simulink model "test_drop_mech"  (Simulink 7.6)
settings: Solver=FixedStepDiscrete  StartTime=0.0  StopTime=0  RelTol=1e-3
undefined symbols (not defined in the file or in its folder): black_al, black_au, black_bl, black_bu, blue_al, blue_au, blue_bl, blue_bu, Down_Camera_Dimensions, gray, green_al, green_au, green_bl, green_bu, Iter_Segment_Thresh, jet, orange_al, orange_au, orange_bl, orange_bu, Rec, red_al, red_au, red_bl, red_bu, Scale_Down_B, Scale_Down_G, Scale_Down_H, Scale_Down_R, Scale_Down_S, Scale_Down_V, SDTV, white_al, white_au, white_bl, white_bu, yellow_al, yellow_au, yellow_bl, yellow_bu
libraries: vipconversions x8, vipgeotforms x6, vipsnks x4, viptextngfix x2, vipsrcs x1
(part 1 of 2)
settings Model: Creator=Thing 1  LastModifiedBy=auvt
settings RTWCC: TargetLang=C++

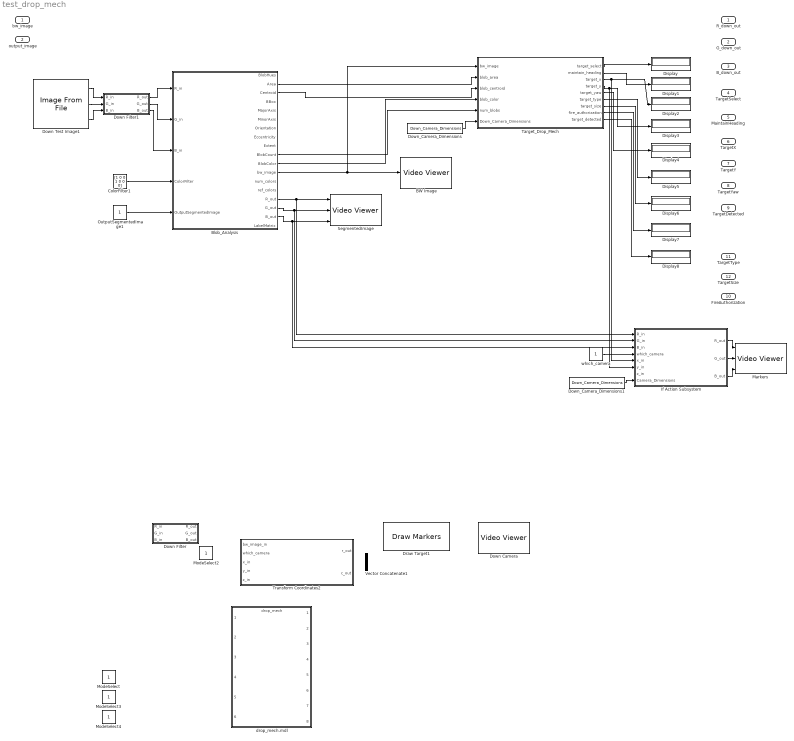
== system test_drop_mech ==
  bw_image : Inport
  output_image : Inport  Port=2
  BW Image : vipsnks/Video Viewer  DialogControllerArgs=DataTag1  inputType=Obsolete7b  imagePorts=One multidimensional signal  useColorMap=off  colormapValue=gray(256)  specRange=off  minInputVal=0  maxInputVal=255  FigPos=[5 861 410 300]  AxisZoom=on  trueSizedOnce=off  OpenAtMdlStart=on
  Blob_Analysis : Subsystem
  ColorFilter1 : Constant  Value=[1 0 0 1 0 0 0]  SampleTime=-1
  Display{,1..8} (9 alike) : Display
  Down Camera : vipsnks/Video Viewer  DialogControllerArgs=DataTag9  inputType=Obsolete7b  imagePorts=Separate color signals  useColorMap=off  colormapValue=jet(256)  specRange=off  minInputVal=0  maxInputVal=255  FigPos=[970 679 274 199]  AxisZoom=on  trueSizedOnce=off  OpenAtMdlStart=on
  Down Filter : Subsystem
  Down Filter1 : Subsystem
  Down Test Image1 : vipsrcs/Image From File  Tag=vipblks_nd  DialogController=vipDDGCreate  DialogControllerArgs=DataTag10  SystemSampleTime=-1  FileName=/home/auvt/auvc/src/vision/Test_Images/drop1.png  imagePorts=Separate color signals  Ts=-1  ImageDataType=double  Signed=on  WordLength=16  sdImageDataType=uint(8)  FractionLengthMode=User-defined  FractionLength=15  OutPortLabels=R|G|B
  Down_Camera_Dimensions : Constant  Value=Down_Camera_Dimensions  SampleTime=-1
  Down_Camera_Dimensions1 : Constant  Value=Down_Camera_Dimensions  SampleTime=-1
  Draw Target1 : viptextngfix/Draw Markers  DialogController=vipDDGCreate  DialogControllerArgs=DataTag11  shape=X-mark  size=7  fill=off  fillClrSource=Specify via dialog  display=User-specified value  intensity=200  color=[0 0 0]  opacity=0.6  viewport=Entire image  antialiasing=off  inType=Obsolete  imagePorts=Separate color signals  prodOutputMode=Binary point scaling  prodOutputWordLength=32  prodOutputFracLength=14  memoryMode=Specify word length  memoryWordLength=16  memoryFracLength=15  roundingMode=Floor  overflowMode=off
  If Action Subsystem : Subsystem  TreatAsAtomicUnit=on
  Markers : vipsnks/Video Viewer  DialogControllerArgs=DataTag14  inputType=Obsolete7b  imagePorts=Separate color signals  useColorMap=off  colormapValue=gray(256)  specRange=off  minInputVal=0  maxInputVal=255  FigPos=[421 436 410 300]  AxisZoom=on  trueSizedOnce=off  OpenAtMdlStart=on
  ModeSelect{,2..4} (4 alike) : Constant  SampleTime=-1
  OutputSegmentedImage1 : Constant  SampleTime=-1
  SegmentedImage : vipsnks/Video Viewer  DialogControllerArgs=DataTag16  inputType=Obsolete7b  imagePorts=Separate color signals  useColorMap=off  colormapValue=gray(256)  specRange=off  minInputVal=0  maxInputVal=255  FigPos=[5 436 410 300]  AxisZoom=on  trueSizedOnce=off  OpenAtMdlStart=on
  Target_Drop_Mech : Stateflow chart  TreatAsAtomicUnit=on  SystemSampleTime=[1/30 0]
  Transform Coordinates2 : Stateflow chart  TreatAsAtomicUnit=on  SystemSampleTime=[1/30 0]
  Vector Concatenate1 : Concatenate  Mode=Multidimensional array
  drop_mech.mdl : ModelReference  ModelNameDialog=drop_mech  SimulationMode=Accelerator  ModelReferenceVersion=1.17  CopyOfModelName=drop_mech
  which_camera : Constant  SampleTime=-1
  R_down_out : Outport  OutDataTypeStr=double
  G_down_out : Outport  Port=2  OutDataTypeStr=double
  B_down_out : Outport  Port=3  OutDataTypeStr=double
  TargetSelect : Outport  Port=4  OutDataTypeStr=double
  MaintainHeading : Outport  Port=5  OutDataTypeStr=double
  TargetX : Outport  Port=6  OutDataTypeStr=double
  TargetY : Outport  Port=7  OutDataTypeStr=double
  TargetYaw : Outport  Port=8  OutDataTypeStr=double
  TargetDetected : Outport  Port=9  OutDataTypeStr=double
  FireAuthorization : Outport  Port=10  OutDataTypeStr=double
  TargetType : Outport  Port=11  OutDataTypeStr=double
  TargetSize : Outport  Port=12  OutDataTypeStr=double
  wires:
  OutputSegmentedImage1/1 -> Blob_Analysis/5(OutputSegmentedImage)
  ColorFilter1/1 -> Blob_Analysis/4(ColorFilter)
  Down Test Image1/1 -> Down Filter1/1(R_in)
  Down Test Image1/2 -> Down Filter1/2(G_in)
  Down Test Image1/3 -> Down Filter1/3(B_in)
  Down Filter1/1(R_out) -> Blob_Analysis/1(R_in)
  Down Filter1/2(G_out) -> Blob_Analysis/2(G_in)
  Down Filter1/3(B_out) -> Blob_Analysis/3(B_in)
  Blob_Analysis/15(R_out) -> If Action Subsystem/1(R_in), SegmentedImage/1
  Blob_Analysis/16(G_out) -> If Action Subsystem/2(G_in), SegmentedImage/2
  Blob_Analysis/17(B_out) -> If Action Subsystem/3(B_in), SegmentedImage/3
  Blob_Analysis/3(Centroid) -> Target_Drop_Mech/3(blob_centroid)
  Blob_Analysis/12(bw_image) -> BW Image/1, Target_Drop_Mech/1(bw_image)
  Blob_Analysis/2(Area) -> Target_Drop_Mech/2(blob_area)
  Blob_Analysis/11(BlobColor) -> Target_Drop_Mech/4(blob_color)
  Blob_Analysis/10(BlobCount) -> Target_Drop_Mech/5(num_blobs)
  Down_Camera_Dimensions/1 -> Target_Drop_Mech/6(Down_Camera_Dimensions)
  Target_Drop_Mech/1(target_select) -> Display/1
  Target_Drop_Mech/2(maintain_heading) -> Display1/1
  Target_Drop_Mech/3(target_x) -> Display2/1, If Action Subsystem/5(x_in)
  Target_Drop_Mech/4(target_y) -> Display3/1, If Action Subsystem/6(y_in)
  Target_Drop_Mech/5(target_yaw) -> Display4/1
  Target_Drop_Mech/6(target_type) -> Display5/1
  Target_Drop_Mech/7(target_size) -> Display6/1
  which_camera/1 -> If Action Subsystem/4(which_camera)
  If Action Subsystem/1(R_out) -> Markers/1
  If Action Subsystem/2(G_out) -> Markers/2
  If Action Subsystem/3(B_out) -> Markers/3
  Down_Camera_Dimensions1/1 -> If Action Subsystem/8(Camera_Dimensions)
  Target_Drop_Mech/8(fire_authorization) -> Display7/1
  Target_Drop_Mech/9(target_detected) -> Display8/1

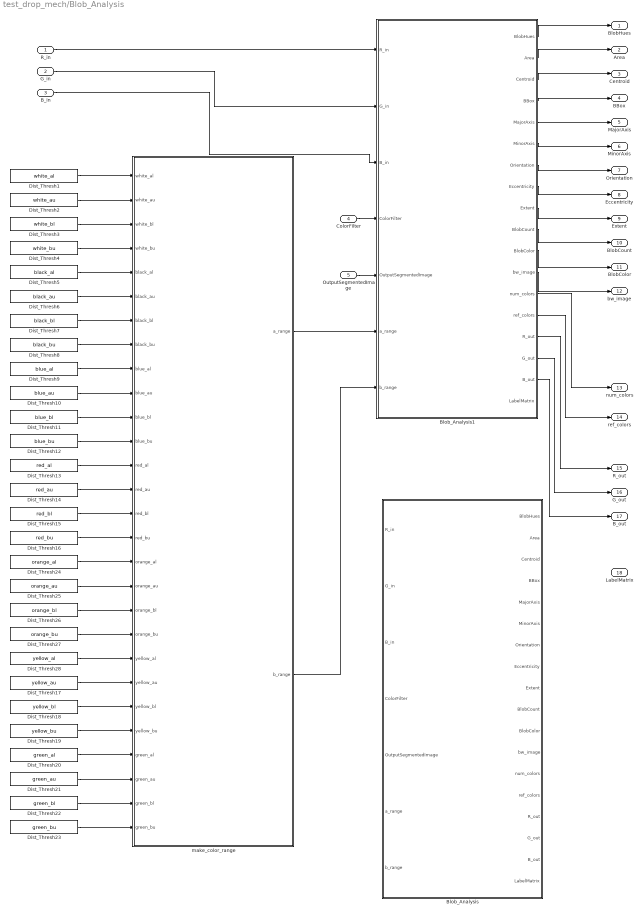
== system test_drop_mech/Blob_Analysis ==
  R_in : Inport
  G_in : Inport  Port=2
  B_in : Inport  Port=3
  ColorFilter : Inport  Port=4
  OutputSegmentedImage : Inport  Port=5
  Blob_Analysis : Subsystem  TreatAsAtomicUnit=on
  Blob_Analysis1 : Subsystem  TreatAsAtomicUnit=on
  Dist_Thresh1 : Constant  Value=white_al  SampleTime=-1
  Dist_Thresh10 : Constant  Value=blue_au  SampleTime=-1
  Dist_Thresh11 : Constant  Value=blue_bl  SampleTime=-1
  Dist_Thresh12 : Constant  Value=blue_bu  SampleTime=-1
  Dist_Thresh13 : Constant  Value=red_al  SampleTime=-1
  Dist_Thresh14 : Constant  Value=red_au  SampleTime=-1
  Dist_Thresh15 : Constant  Value=red_bl  SampleTime=-1
  Dist_Thresh16 : Constant  Value=red_bu  SampleTime=-1
  Dist_Thresh17 : Constant  Value=yellow_au  SampleTime=-1
  Dist_Thresh18 : Constant  Value=yellow_bl  SampleTime=-1
  Dist_Thresh19 : Constant  Value=yellow_bu  SampleTime=-1
  Dist_Thresh2 : Constant  Value=white_au  SampleTime=-1
  Dist_Thresh20 : Constant  Value=green_al  SampleTime=-1
  Dist_Thresh21 : Constant  Value=green_au  SampleTime=-1
  Dist_Thresh22 : Constant  Value=green_bl  SampleTime=-1
  Dist_Thresh23 : Constant  Value=green_bu  SampleTime=-1
  Dist_Thresh24 : Constant  Value=orange_al  SampleTime=-1
  Dist_Thresh25 : Constant  Value=orange_au  SampleTime=-1
  Dist_Thresh26 : Constant  Value=orange_bl  SampleTime=-1
  Dist_Thresh27 : Constant  Value=orange_bu  SampleTime=-1
  Dist_Thresh28 : Constant  Value=yellow_al  SampleTime=-1
  Dist_Thresh3 : Constant  Value=white_bl  SampleTime=-1
  Dist_Thresh4 : Constant  Value=white_bu  SampleTime=-1
  Dist_Thresh5 : Constant  Value=black_al  SampleTime=-1
  Dist_Thresh6 : Constant  Value=black_au  SampleTime=-1
  Dist_Thresh7 : Constant  Value=black_bl  SampleTime=-1
  Dist_Thresh8 : Constant  Value=black_bu  SampleTime=-1
  Dist_Thresh9 : Constant  Value=blue_al  SampleTime=-1
  make_color_range : Stateflow chart  TreatAsAtomicUnit=on
  BlobHues : Outport
  Area : Outport  Port=2
  Centroid : Outport  Port=3
  BBox : Outport  Port=4
  MajorAxis : Outport  Port=5
  MinorAxis : Outport  Port=6
  Orientation : Outport  Port=7
  Eccentricity : Outport  Port=8
  Extent : Outport  Port=9
  BlobCount : Outport  Port=10
  BlobColor : Outport  Port=11
  bw_image : Outport  Port=12
  num_colors : Outport  Port=13
  ref_colors : Outport  Port=14
  R_out : Outport  Port=15
  G_out : Outport  Port=16
  B_out : Outport  Port=17
  LabelMatrix : Outport  Port=18
  wires:
  ColorFilter/1 -> Blob_Analysis1/4(ColorFilter)
  OutputSegmentedImage/1 -> Blob_Analysis1/5(OutputSegmentedImage)
  make_color_range/2(b_range) -> Blob_Analysis1/7(b_range)
  make_color_range/1(a_range) -> Blob_Analysis1/6(a_range)
  B_in/1 -> Blob_Analysis1/3(B_in)
  G_in/1 -> Blob_Analysis1/2(G_in)
  R_in/1 -> Blob_Analysis1/1(R_in)
  Dist_Thresh7/1 -> make_color_range/7(black_bl)
  Dist_Thresh6/1 -> make_color_range/6(black_au)
  Dist_Thresh5/1 -> make_color_range/5(black_al)
  Dist_Thresh4/1 -> make_color_range/4(white_bu)
  Dist_Thresh3/1 -> make_color_range/3(white_bl)
  Dist_Thresh2/1 -> make_color_range/2(white_au)
  Dist_Thresh8/1 -> make_color_range/8(black_bu)
  Dist_Thresh9/1 -> make_color_range/9(blue_al)
  Dist_Thresh10/1 -> make_color_range/10(blue_au)
  Dist_Thresh11/1 -> make_color_range/11(blue_bl)
  Dist_Thresh12/1 -> make_color_range/12(blue_bu)
  Dist_Thresh13/1 -> make_color_range/13(red_al)
  Dist_Thresh14/1 -> make_color_range/14(red_au)
  Dist_Thresh15/1 -> make_color_range/15(red_bl)
  Dist_Thresh16/1 -> make_color_range/16(red_bu)
  Dist_Thresh24/1 -> make_color_range/17(orange_al)
  Dist_Thresh25/1 -> make_color_range/18(orange_au)
  Dist_Thresh26/1 -> make_color_range/19(orange_bl)
  Dist_Thresh27/1 -> make_color_range/20(orange_bu)
  Dist_Thresh21/1 -> make_color_range/26(green_au)
  Dist_Thresh28/1 -> make_color_range/21(yellow_al)
  Dist_Thresh17/1 -> make_color_range/22(yellow_au)
  Dist_Thresh20/1 -> make_color_range/25(green_al)
  Dist_Thresh19/1 -> make_color_range/24(yellow_bu)
  Dist_Thresh18/1 -> make_color_range/23(yellow_bl)
  Dist_Thresh1/1 -> make_color_range/1(white_al)
  Dist_Thresh22/1 -> make_color_range/27(green_bl)
  Dist_Thresh23/1 -> make_color_range/28(green_bu)
  Blob_Analysis1/1(BlobHues) -> BlobHues/1
  Blob_Analysis1/2(Area) -> Area/1
  Blob_Analysis1/3(Centroid) -> Centroid/1
  Blob_Analysis1/4(BBox) -> BBox/1
  Blob_Analysis1/5(MajorAxis) -> MajorAxis/1
  Blob_Analysis1/6(MinorAxis) -> MinorAxis/1
  Blob_Analysis1/7(Orientation) -> Orientation/1
  Blob_Analysis1/8(Eccentricity) -> Eccentricity/1
  Blob_Analysis1/9(Extent) -> Extent/1
  Blob_Analysis1/10(BlobCount) -> BlobCount/1
  Blob_Analysis1/11(BlobColor) -> BlobColor/1
  Blob_Analysis1/12(bw_image) -> bw_image/1
  Blob_Analysis1/13(num_colors) -> num_colors/1
  Blob_Analysis1/14(ref_colors) -> ref_colors/1
  Blob_Analysis1/15(R_out) -> R_out/1
  Blob_Analysis1/16(G_out) -> G_out/1
  Blob_Analysis1/17(B_out) -> B_out/1

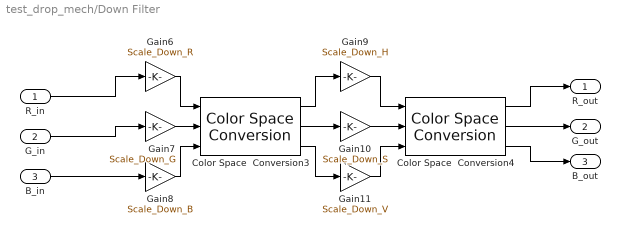
== system test_drop_mech/Down Filter ==
  R_in : Inport  PortDimensions=Down_Camera_Dimensions
  G_in : Inport  Port=2  PortDimensions=Down_Camera_Dimensions
  B_in : Inport  Port=3  PortDimensions=Down_Camera_Dimensions
  Color Space  Conversion3 : vipconversions/Color Space  Conversion  conversion=Obsolete  conversionActive=R'G'B' to HSV  wp_str=D50  rec=Rec. 601 (SDTV)  sys=1125/60/2:1  imagePorts=Separate color signals
  Color Space  Conversion4 : vipconversions/Color Space  Conversion  conversion=Obsolete  conversionActive=HSV to R'G'B'  wp_str=D50  rec=Rec. 601 (SDTV)  sys=1125/60/2:1  imagePorts=Separate color signals
  Gain10 : Gain  Gain=Scale_Down_S
  Gain11 : Gain  Gain=Scale_Down_V
  Gain6 : Gain  Gain=Scale_Down_R
  Gain7 : Gain  Gain=Scale_Down_G
  Gain8 : Gain  Gain=Scale_Down_B
  Gain9 : Gain  Gain=Scale_Down_H
  R_out : Outport  OutDataTypeStr=double
  G_out : Outport  Port=2  OutDataTypeStr=double
  B_out : Outport  Port=3  OutDataTypeStr=double
  wires:
  Gain6/1 -> Color Space  Conversion3/1
  Gain7/1 -> Color Space  Conversion3/2
  Gain8/1 -> Color Space  Conversion3/3
  Color Space  Conversion3/1 -> Gain9/1
  Color Space  Conversion3/2 -> Gain10/1
  Color Space  Conversion3/3 -> Gain11/1
  Gain9/1 -> Color Space  Conversion4/1
  Gain10/1 -> Color Space  Conversion4/2
  Gain11/1 -> Color Space  Conversion4/3
  R_in/1 -> Gain6/1
  G_in/1 -> Gain7/1
  B_in/1 -> Gain8/1
  Color Space  Conversion4/1 -> R_out/1
  Color Space  Conversion4/2 -> G_out/1
  Color Space  Conversion4/3 -> B_out/1

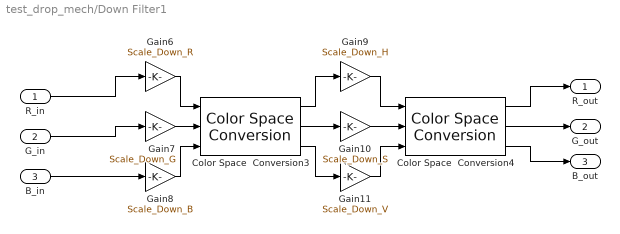
== system test_drop_mech/Down Filter1 ==
  R_in : Inport  PortDimensions=Down_Camera_Dimensions
  G_in : Inport  Port=2  PortDimensions=Down_Camera_Dimensions
  B_in : Inport  Port=3  PortDimensions=Down_Camera_Dimensions
  Color Space  Conversion3 : vipconversions/Color Space  Conversion  conversion=Obsolete  conversionActive=R'G'B' to HSV  wp_str=D50  rec=Rec. 601 (SDTV)  sys=1125/60/2:1  imagePorts=Separate color signals
  Color Space  Conversion4 : vipconversions/Color Space  Conversion  conversion=Obsolete  conversionActive=HSV to R'G'B'  wp_str=D50  rec=Rec. 601 (SDTV)  sys=1125/60/2:1  imagePorts=Separate color signals
  Gain10 : Gain  Gain=Scale_Down_S
  Gain11 : Gain  Gain=Scale_Down_V
  Gain6 : Gain  Gain=Scale_Down_R
  Gain7 : Gain  Gain=Scale_Down_G
  Gain8 : Gain  Gain=Scale_Down_B
  Gain9 : Gain  Gain=Scale_Down_H
  R_out : Outport  OutDataTypeStr=double
  G_out : Outport  Port=2  OutDataTypeStr=double
  B_out : Outport  Port=3  OutDataTypeStr=double
  wires:
  Gain6/1 -> Color Space  Conversion3/1
  Gain7/1 -> Color Space  Conversion3/2
  Gain8/1 -> Color Space  Conversion3/3
  Color Space  Conversion3/1 -> Gain9/1
  Color Space  Conversion3/2 -> Gain10/1
  Color Space  Conversion3/3 -> Gain11/1
  Gain9/1 -> Color Space  Conversion4/1
  Gain10/1 -> Color Space  Conversion4/2
  Gain11/1 -> Color Space  Conversion4/3
  R_in/1 -> Gain6/1
  G_in/1 -> Gain7/1
  B_in/1 -> Gain8/1
  Color Space  Conversion4/1 -> R_out/1
  Color Space  Conversion4/2 -> G_out/1
  Color Space  Conversion4/3 -> B_out/1

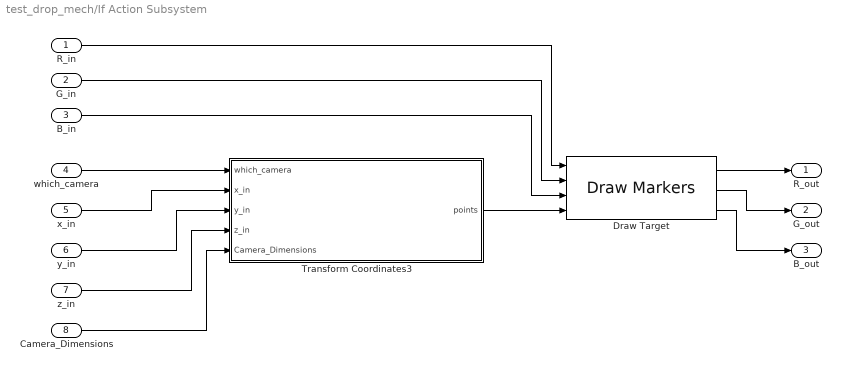
== system test_drop_mech/If Action Subsystem ==
  R_in : Inport
  G_in : Inport  Port=2
  B_in : Inport  Port=3
  which_camera : Inport  Port=4
  x_in : Inport  Port=5
  y_in : Inport  Port=6
  z_in : Inport  Port=7
  Camera_Dimensions : Inport  Port=8
  Draw Target : viptextngfix/Draw Markers  DialogController=vipDDGCreate  DialogControllerArgs=DataTag12  shape=X-mark  size=7  fill=off  fillClrSource=Specify via dialog  display=User-specified value  intensity=200  color=[1 1 0]  opacity=0.6  viewport=Entire image  antialiasing=off  inType=Obsolete  imagePorts=Separate color signals  prodOutputMode=Binary point scaling  prodOutputWordLength=32  prodOutputFracLength=14  memoryMode=Specify word length  memoryWordLength=16  memoryFracLength=15  roundingMode=Floor  overflowMode=off
  Transform Coordinates3 : Stateflow chart  TreatAsAtomicUnit=on
  R_out : Outport  OutDataTypeStr=double
  G_out : Outport  Port=2  OutDataTypeStr=double
  B_out : Outport  Port=3  OutDataTypeStr=double
  wires:
  which_camera/1 -> Transform Coordinates3/1(which_camera)
  x_in/1 -> Transform Coordinates3/2(x_in)
  y_in/1 -> Transform Coordinates3/3(y_in)
  z_in/1 -> Transform Coordinates3/4(z_in)
  Camera_Dimensions/1 -> Transform Coordinates3/5(Camera_Dimensions)
  Draw Target/1 -> R_out/1
  Draw Target/2 -> G_out/1
  Draw Target/3 -> B_out/1
  R_in/1 -> Draw Target/1
  G_in/1 -> Draw Target/2
  B_in/1 -> Draw Target/3
  Transform Coordinates3/1(points) -> Draw Target/4

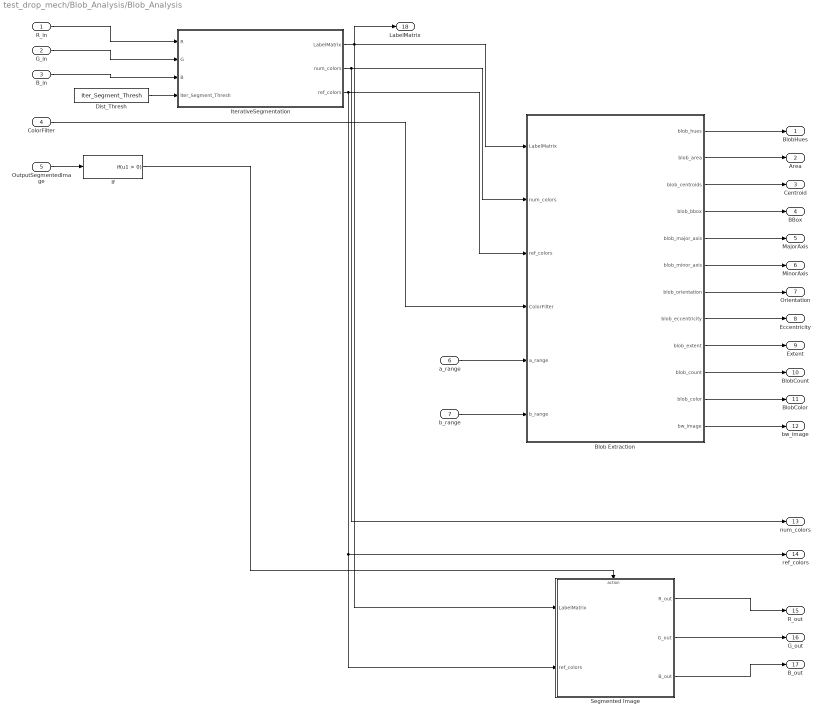
== system test_drop_mech/Blob_Analysis/Blob_Analysis ==
  R_in : Inport
  G_in : Inport  Port=2
  B_in : Inport  Port=3
  ColorFilter : Inport  Port=4
  OutputSegmentedImage : Inport  Port=5
  a_range : Inport  Port=6
  b_range : Inport  Port=7
  Blob Extraction : Stateflow chart  TreatAsAtomicUnit=on
  Dist_Thresh : Constant  Value=Iter_Segment_Thresh  SampleTime=-1
  If : If  ShowElse=off
  IterativeSegmentation : Subsystem
      settings: UndoDeleteFcn=Stateflow.SLINSF.SimulinkMan.restorePreDeleteFcn  PreDeleteFcn=Stateflow.SLINSF.SimulinkMan.removePreDeleteFcn
  Segmented Image : Subsystem  TreatAsAtomicUnit=on
  BlobHues : Outport
  Area : Outport  Port=2
  Centroid : Outport  Port=3
  BBox : Outport  Port=4
  MajorAxis : Outport  Port=5
  MinorAxis : Outport  Port=6
  Orientation : Outport  Port=7
  Eccentricity : Outport  Port=8
  Extent : Outport  Port=9
  BlobCount : Outport  Port=10
  BlobColor : Outport  Port=11
  bw_image : Outport  Port=12
  num_colors : Outport  Port=13
  ref_colors : Outport  Port=14
  R_out : Outport  Port=15
  G_out : Outport  Port=16
  B_out : Outport  Port=17
  LabelMatrix : Outport  Port=18
  wires:
  Blob Extraction/11(blob_color) -> BlobColor/1
  Segmented Image/3(B_out) -> B_out/1
  Segmented Image/2(G_out) -> G_out/1
  Segmented Image/1(R_out) -> R_out/1
  OutputSegmentedImage/1 -> If/1
  If/1 -> Segmented Image/Action
  B_in/1 -> IterativeSegmentation/3(B)
  G_in/1 -> IterativeSegmentation/2(G)
  R_in/1 -> IterativeSegmentation/1(R)
  Dist_Thresh/1 -> IterativeSegmentation/4(Iter_Segment_Thresh)
  IterativeSegmentation/3(ref_colors) -> ref_colors/1, Segmented Image/2(ref_colors), Blob Extraction/3(ref_colors)
  IterativeSegmentation/2(num_colors) -> num_colors/1, Blob Extraction/2(num_colors)
  IterativeSegmentation/1(LabelMatrix) -> LabelMatrix/1, Segmented Image/1(LabelMatrix), Blob Extraction/1(LabelMatrix)
  b_range/1 -> Blob Extraction/6(b_range)
  a_range/1 -> Blob Extraction/5(a_range)
  ColorFilter/1 -> Blob Extraction/4(ColorFilter)
  Blob Extraction/1(blob_hues) -> BlobHues/1
  Blob Extraction/2(blob_area) -> Area/1
  Blob Extraction/3(blob_centroids) -> Centroid/1
  Blob Extraction/4(blob_bbox) -> BBox/1
  Blob Extraction/5(blob_major_axis) -> MajorAxis/1
  Blob Extraction/6(blob_minor_axis) -> MinorAxis/1
  Blob Extraction/7(blob_orientation) -> Orientation/1
  Blob Extraction/8(blob_eccentricity) -> Eccentricity/1
  Blob Extraction/9(blob_extent) -> Extent/1
  Blob Extraction/10(blob_count) -> BlobCount/1
  Blob Extraction/12(bw_image) -> bw_image/1

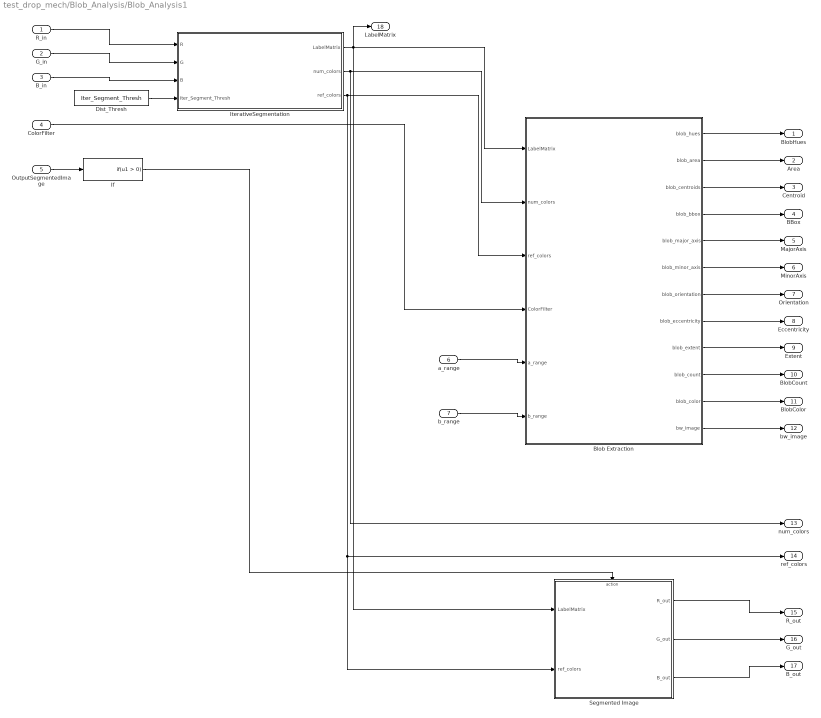
== system test_drop_mech/Blob_Analysis/Blob_Analysis1 ==
  R_in : Inport
  G_in : Inport  Port=2
  B_in : Inport  Port=3
  ColorFilter : Inport  Port=4
  OutputSegmentedImage : Inport  Port=5
  a_range : Inport  Port=6
  b_range : Inport  Port=7
  Blob Extraction : Stateflow chart  TreatAsAtomicUnit=on
  Dist_Thresh : Constant  Value=Iter_Segment_Thresh  SampleTime=-1
  If : If  ShowElse=off
  IterativeSegmentation : Subsystem
      settings: UndoDeleteFcn=Stateflow.SLINSF.SimulinkMan.restorePreDeleteFcn  PreDeleteFcn=Stateflow.SLINSF.SimulinkMan.removePreDeleteFcn
  Segmented Image : Subsystem  TreatAsAtomicUnit=on
  BlobHues : Outport
  Area : Outport  Port=2
  Centroid : Outport  Port=3
  BBox : Outport  Port=4
  MajorAxis : Outport  Port=5
  MinorAxis : Outport  Port=6
  Orientation : Outport  Port=7
  Eccentricity : Outport  Port=8
  Extent : Outport  Port=9
  BlobCount : Outport  Port=10
  BlobColor : Outport  Port=11
  bw_image : Outport  Port=12
  num_colors : Outport  Port=13
  ref_colors : Outport  Port=14
  R_out : Outport  Port=15
  G_out : Outport  Port=16
  B_out : Outport  Port=17
  LabelMatrix : Outport  Port=18
  wires:
  Blob Extraction/12(bw_image) -> bw_image/1
  Blob Extraction/10(blob_count) -> BlobCount/1
  Blob Extraction/9(blob_extent) -> Extent/1
  Blob Extraction/8(blob_eccentricity) -> Eccentricity/1
  Blob Extraction/7(blob_orientation) -> Orientation/1
  Blob Extraction/6(blob_minor_axis) -> MinorAxis/1
  Blob Extraction/5(blob_major_axis) -> MajorAxis/1
  Blob Extraction/4(blob_bbox) -> BBox/1
  Blob Extraction/3(blob_centroids) -> Centroid/1
  Blob Extraction/2(blob_area) -> Area/1
  Blob Extraction/1(blob_hues) -> BlobHues/1
  ColorFilter/1 -> Blob Extraction/4(ColorFilter)
  a_range/1 -> Blob Extraction/5(a_range)
  b_range/1 -> Blob Extraction/6(b_range)
  IterativeSegmentation/1(LabelMatrix) -> Blob Extraction/1(LabelMatrix), Segmented Image/1(LabelMatrix), LabelMatrix/1
  IterativeSegmentation/2(num_colors) -> Blob Extraction/2(num_colors), num_colors/1
  IterativeSegmentation/3(ref_colors) -> Blob Extraction/3(ref_colors), Segmented Image/2(ref_colors), ref_colors/1
  Dist_Thresh/1 -> IterativeSegmentation/4(Iter_Segment_Thresh)
  R_in/1 -> IterativeSegmentation/1(R)
  G_in/1 -> IterativeSegmentation/2(G)
  B_in/1 -> IterativeSegmentation/3(B)
  If/1 -> Segmented Image/Action
  OutputSegmentedImage/1 -> If/1
  Segmented Image/1(R_out) -> R_out/1
  Segmented Image/2(G_out) -> G_out/1
  Segmented Image/3(B_out) -> B_out/1
  Blob Extraction/11(blob_color) -> BlobColor/1

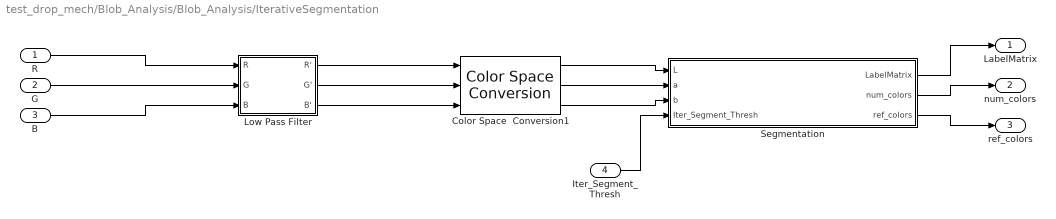
== system test_drop_mech/Blob_Analysis/Blob_Analysis/IterativeSegmentation ==
  R : Inport
  G : Inport  Port=2
  B : Inport  Port=3
  Iter_Segment_Thresh : Inport  Port=4
  Color Space  Conversion1 : vipconversions/Color Space  Conversion  conversion=Obsolete  conversionActive=sR'G'B' to L*a*b*  wp_str=D50  rec=Rec. 601 (SDTV)  sys=1125/60/2:1  imagePorts=Separate color signals
  Low Pass Filter : Subsystem
  Segmentation : Subsystem
  LabelMatrix : Outport
  num_colors : Outport  Port=2
  ref_colors : Outport  Port=3
  wires:
  Iter_Segment_Thresh/1 -> Segmentation/4(Iter_Segment_Thresh)
  Segmentation/3(ref_colors) -> ref_colors/1
  Segmentation/2(num_colors) -> num_colors/1
  Segmentation/1(LabelMatrix) -> LabelMatrix/1
  B/1 -> Low Pass Filter/3(B)
  G/1 -> Low Pass Filter/2(G)
  R/1 -> Low Pass Filter/1(R)
  Color Space  Conversion1/1 -> Segmentation/1(L)
  Color Space  Conversion1/2 -> Segmentation/2(a)
  Color Space  Conversion1/3 -> Segmentation/3(b)
  Low Pass Filter/1(R') -> Color Space  Conversion1/1
  Low Pass Filter/2(G') -> Color Space  Conversion1/2
  Low Pass Filter/3(B') -> Color Space  Conversion1/3

== system test_drop_mech/Blob_Analysis/Blob_Analysis/Segmented Image ==
  LabelMatrix : Inport
  ref_colors : Inport  Port=2
  Action Port : ActionPort
  Color Space  Conversion : vipconversions/Color Space  Conversion  conversion=Obsolete  conversionActive=L*a*b* to sR'G'B'  wp_str=D65  rec=Rec. 601 (SDTV)  sys=1125/60/2:1  imagePorts=Separate color signals
  Display Image : Stateflow chart  TreatAsAtomicUnit=on
  R_out : Outport
  G_out : Outport  Port=2
  B_out : Outport  Port=3
  wires:
  Color Space  Conversion/3 -> B_out/1
  Color Space  Conversion/2 -> G_out/1
  Color Space  Conversion/1 -> R_out/1
  Display Image/3(b) -> Color Space  Conversion/3
  Display Image/2(a) -> Color Space  Conversion/2
  Display Image/1(L) -> Color Space  Conversion/1
  ref_colors/1 -> Display Image/2(ref_colors)
  LabelMatrix/1 -> Display Image/1(LabelMatrix)

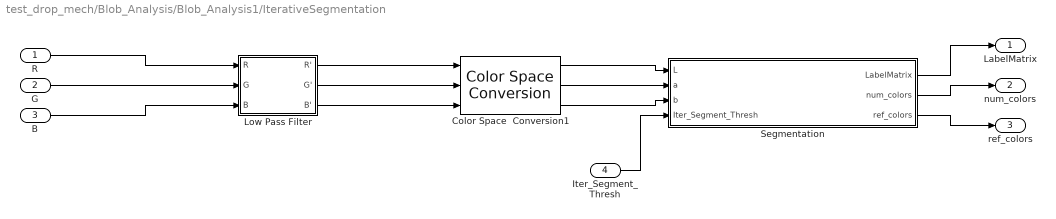
== system test_drop_mech/Blob_Analysis/Blob_Analysis1/IterativeSegmentation ==
  R : Inport
  G : Inport  Port=2
  B : Inport  Port=3
  Iter_Segment_Thresh : Inport  Port=4
  Color Space  Conversion1 : vipconversions/Color Space  Conversion  conversion=Obsolete  conversionActive=sR'G'B' to L*a*b*  wp_str=D50  rec=Rec. 601 (SDTV)  sys=1125/60/2:1  imagePorts=Separate color signals
  Low Pass Filter : Subsystem
  Segmentation : Subsystem
  LabelMatrix : Outport
  num_colors : Outport  Port=2
  ref_colors : Outport  Port=3
  wires:
  Low Pass Filter/3(B') -> Color Space  Conversion1/3
  Low Pass Filter/2(G') -> Color Space  Conversion1/2
  Low Pass Filter/1(R') -> Color Space  Conversion1/1
  Color Space  Conversion1/3 -> Segmentation/3(b)
  Color Space  Conversion1/2 -> Segmentation/2(a)
  Color Space  Conversion1/1 -> Segmentation/1(L)
  R/1 -> Low Pass Filter/1(R)
  G/1 -> Low Pass Filter/2(G)
  B/1 -> Low Pass Filter/3(B)
  Segmentation/1(LabelMatrix) -> LabelMatrix/1
  Segmentation/2(num_colors) -> num_colors/1
  Segmentation/3(ref_colors) -> ref_colors/1
  Iter_Segment_Thresh/1 -> Segmentation/4(Iter_Segment_Thresh)

== system test_drop_mech/Blob_Analysis/Blob_Analysis1/Segmented Image ==
  LabelMatrix : Inport
  ref_colors : Inport  Port=2
  Action Port : ActionPort  ActionType=then
  Color Space  Conversion : vipconversions/Color Space  Conversion  conversion=Obsolete  conversionActive=L*a*b* to sR'G'B'  wp_str=D65  rec=Rec. 601 (SDTV)  sys=1125/60/2:1  imagePorts=Separate color signals
  Display Image : Stateflow chart  TreatAsAtomicUnit=on
  R_out : Outport
  G_out : Outport  Port=2
  B_out : Outport  Port=3
  wires:
  LabelMatrix/1 -> Display Image/1(LabelMatrix)
  ref_colors/1 -> Display Image/2(ref_colors)
  Display Image/1(L) -> Color Space  Conversion/1
  Display Image/2(a) -> Color Space  Conversion/2
  Display Image/3(b) -> Color Space  Conversion/3
  Color Space  Conversion/1 -> R_out/1
  Color Space  Conversion/2 -> G_out/1
  Color Space  Conversion/3 -> B_out/1

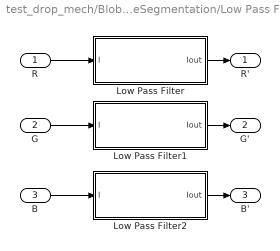
== system test_drop_mech/Blob_Analysis/Blob_Analysis/IterativeSegmentation/Low Pass Filter ==
  R : Inport
  G : Inport  Port=2
  B : Inport  Port=3
  Low Pass Filter : Stateflow chart  TreatAsAtomicUnit=on
  Low Pass Filter1 : Stateflow chart  TreatAsAtomicUnit=on
  Low Pass Filter2 : Stateflow chart  TreatAsAtomicUnit=on
  R' : Outport
  G' : Outport  Port=2
  B' : Outport  Port=3
  wires:
  R/1 -> Low Pass Filter/1(I)
  G/1 -> Low Pass Filter1/1(I)
  B/1 -> Low Pass Filter2/1(I)
  Low Pass Filter1/1(Iout) -> G'/1
  Low Pass Filter2/1(Iout) -> B'/1
  Low Pass Filter/1(Iout) -> R'/1

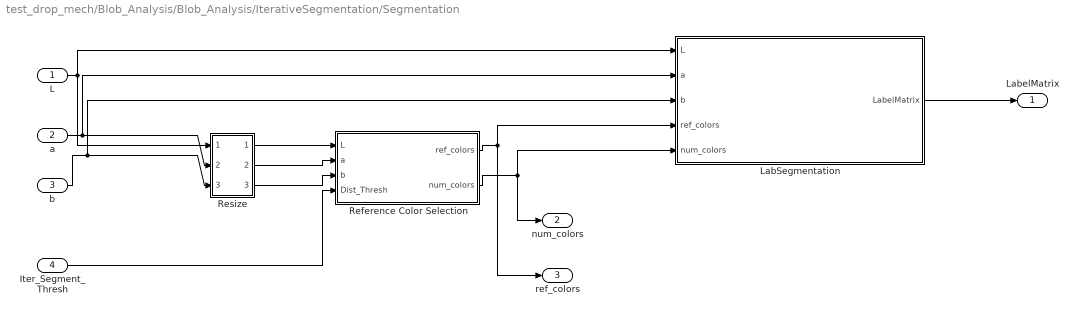
== system test_drop_mech/Blob_Analysis/Blob_Analysis/IterativeSegmentation/Segmentation ==
  L : Inport
  a : Inport  Port=2
  b : Inport  Port=3
  Iter_Segment_Thresh : Inport  Port=4
  LabSegmentation : Stateflow chart  TreatAsAtomicUnit=on
  Reference Color Selection : Stateflow chart  TreatAsAtomicUnit=on
  Resize : Subsystem
  LabelMatrix : Outport
  num_colors : Outport  Port=2
  ref_colors : Outport  Port=3
  wires:
  L/1 -> Resize/1(In1), LabSegmentation/1(L)
  a/1 -> Resize/2(In2), LabSegmentation/2(a)
  b/1 -> Resize/3(In3), LabSegmentation/3(b)
  Resize/1(Out1) -> Reference Color Selection/1(L)
  Resize/2(Out2) -> Reference Color Selection/2(a)
  Resize/3(Out3) -> Reference Color Selection/3(b)
  Reference Color Selection/1(ref_colors) -> LabSegmentation/4(ref_colors), ref_colors/1
  Reference Color Selection/2(num_colors) -> num_colors/1, LabSegmentation/5(num_colors)
  LabSegmentation/1(LabelMatrix) -> LabelMatrix/1
  Iter_Segment_Thresh/1 -> Reference Color Selection/4(Dist_Thresh)

== system test_drop_mech/Blob_Analysis/Blob_Analysis1/IterativeSegmentation/Low Pass Filter ==
  R : Inport
  G : Inport  Port=2
  B : Inport  Port=3
  Low Pass Filter : Stateflow chart  TreatAsAtomicUnit=on
  Low Pass Filter1 : Stateflow chart  TreatAsAtomicUnit=on
  Low Pass Filter2 : Stateflow chart  TreatAsAtomicUnit=on
  R' : Outport
  G' : Outport  Port=2
  B' : Outport  Port=3
  wires:
  Low Pass Filter/1(Iout) -> R'/1
  Low Pass Filter2/1(Iout) -> B'/1
  Low Pass Filter1/1(Iout) -> G'/1
  B/1 -> Low Pass Filter2/1(I)
  G/1 -> Low Pass Filter1/1(I)
  R/1 -> Low Pass Filter/1(I)

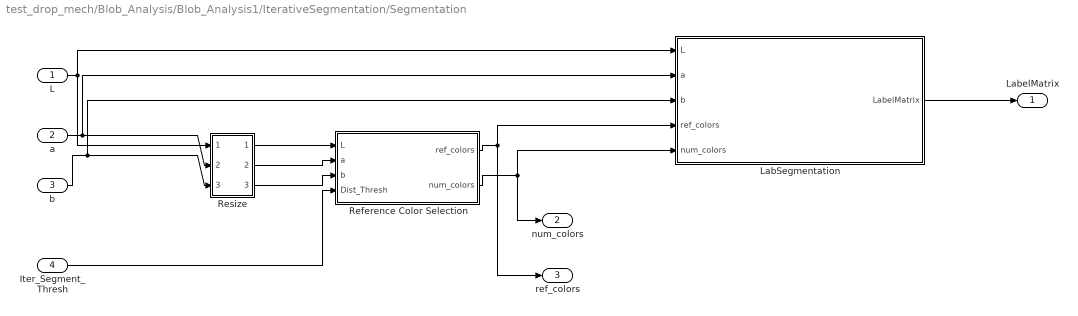
== system test_drop_mech/Blob_Analysis/Blob_Analysis1/IterativeSegmentation/Segmentation ==
  L : Inport
  a : Inport  Port=2
  b : Inport  Port=3
  Iter_Segment_Thresh : Inport  Port=4
  LabSegmentation : Stateflow chart  TreatAsAtomicUnit=on
  Reference Color Selection : Stateflow chart  TreatAsAtomicUnit=on
  Resize : Subsystem
  LabelMatrix : Outport
  num_colors : Outport  Port=2
  ref_colors : Outport  Port=3
  wires:
  Iter_Segment_Thresh/1 -> Reference Color Selection/4(Dist_Thresh)
  LabSegmentation/1(LabelMatrix) -> LabelMatrix/1
  Reference Color Selection/2(num_colors) -> LabSegmentation/5(num_colors), num_colors/1
  Reference Color Selection/1(ref_colors) -> ref_colors/1, LabSegmentation/4(ref_colors)
  Resize/3(Out3) -> Reference Color Selection/3(b)
  Resize/2(Out2) -> Reference Color Selection/2(a)
  Resize/1(Out1) -> Reference Color Selection/1(L)
  b/1 -> LabSegmentation/3(b), Resize/3(In3)
  a/1 -> LabSegmentation/2(a), Resize/2(In2)
  L/1 -> LabSegmentation/1(L), Resize/1(In1)

== system test_drop_mech/Blob_Analysis/Blob_Analysis/IterativeSegmentation/Segmentation/Resize ==
  In1 : Inport
  In2 : Inport  Port=2
  In3 : Inport  Port=3
  Resize : vipgeotforms/Resize  DialogController=vipDDGCreate  DialogControllerArgs=DataTag2  specify=Number of output rows and columns  rfactor=[]  outCols=25  outRows=25  outRowsCols=[60 80]  interp_method=Bilinear  antialias=on  useROI=off  roiFlag=off  prodOutputMode=Binary point scaling  prodOutputWordLength=32  prodOutputFracLength=10  roundingMode=Nearest  overflowMode=on
  Resize1 : vipgeotforms/Resize  DialogController=vipDDGCreate  DialogControllerArgs=DataTag3  specify=Number of output rows and columns  rfactor=[200 150]  outCols=25  outRows=25  outRowsCols=[60 80]  interp_method=Bilinear  antialias=on  useROI=off  roiFlag=off  prodOutputMode=Binary point scaling  prodOutputWordLength=32  prodOutputFracLength=10  roundingMode=Nearest  overflowMode=on
  Resize2 : vipgeotforms/Resize  DialogController=vipDDGCreate  DialogControllerArgs=DataTag4  specify=Number of output rows and columns  rfactor=[200 150]  outCols=25  outRows=25  outRowsCols=[60 80]  interp_method=Bilinear  antialias=on  useROI=off  roiFlag=off  prodOutputMode=Binary point scaling  prodOutputWordLength=32  prodOutputFracLength=10  roundingMode=Nearest  overflowMode=on
  Out1 : Outport
  Out2 : Outport  Port=2
  Out3 : Outport  Port=3
  wires:
  In1/1 -> Resize/1
  Resize/1 -> Out1/1
  In2/1 -> Resize1/1
  Resize1/1 -> Out2/1
  In3/1 -> Resize2/1
  Resize2/1 -> Out3/1

== system test_drop_mech/Blob_Analysis/Blob_Analysis1/IterativeSegmentation/Segmentation/Resize ==
  In1 : Inport
  In2 : Inport  Port=2
  In3 : Inport  Port=3
  Resize : vipgeotforms/Resize  DialogController=vipDDGCreate  DialogControllerArgs=DataTag5  specify=Number of output rows and columns  rfactor=[]  outCols=25  outRows=25  outRowsCols=[60 80]  interp_method=Bilinear  antialias=on  useROI=off  roiFlag=off  prodOutputMode=Binary point scaling  prodOutputWordLength=32  prodOutputFracLength=10  roundingMode=Nearest  overflowMode=on
  Resize1 : vipgeotforms/Resize  DialogController=vipDDGCreate  DialogControllerArgs=DataTag6  specify=Number of output rows and columns  rfactor=[200 150]  outCols=25  outRows=25  outRowsCols=[60 80]  interp_method=Bilinear  antialias=on  useROI=off  roiFlag=off  prodOutputMode=Binary point scaling  prodOutputWordLength=32  prodOutputFracLength=10  roundingMode=Nearest  overflowMode=on
  Resize2 : vipgeotforms/Resize  DialogController=vipDDGCreate  DialogControllerArgs=DataTag7  specify=Number of output rows and columns  rfactor=[200 150]  outCols=25  outRows=25  outRowsCols=[60 80]  interp_method=Bilinear  antialias=on  useROI=off  roiFlag=off  prodOutputMode=Binary point scaling  prodOutputWordLength=32  prodOutputFracLength=10  roundingMode=Nearest  overflowMode=on
  Out1 : Outport
  Out2 : Outport  Port=2
  Out3 : Outport  Port=3
  wires:
  Resize2/1 -> Out3/1
  In3/1 -> Resize2/1
  Resize1/1 -> Out2/1
  In2/1 -> Resize1/1
  Resize/1 -> Out1/1
  In1/1 -> Resize/1

== matlab function If Action Subsystem/Transform Coordinates3 ==
  data: which_camera input double; x_in input double; y_in input double; z_in input double; Camera_Dimensions input double; points output double
function points = transform_G2L(which_camera, x_in, y_in, z_in, Camera_Dimensions)
% This function, "transform Global to Local coordinates," transforms
%   global coordinates that are sent to the controller into local
%   coordinates that can be displayed over images.
%
% 5-29-11
%
% Input
%   x_in, y_in, z_in = vectors of points in global (vehicle-centered)
%     coordinate system
%   bw_image_in = a 2-D array of pixel values (used only to extract image
%     size)
%   which_camera = selects which camera for relative coordinates
%                = 0 -> Forward camera
%                = 1 -> Down camera
%
% Output
%   r_out, c_out = row, column pairs in local coordinate system

rows = Camera_Dimensions(1);
cols = Camera_Dimensions(2);
if( which_camera == 0 )
    points = [z_in + floor(rows/2);
              y_in + floor(cols/2)];
else
    points = [floor(rows/2) - x_in;
              y_in + floor(cols/2)];
end


return

== matlab function Blob_Analysis/Blob_Analysis1/Blob Extraction ==
  data: LabelMatrix input double; num_colors input double; ref_colors input double; ColorFilter input double; a_range input double; b_range input double; blob_hues output double; blob_area output double; blob_centroids output double; blob_bbox output double; blob_major_axis output double; blob_minor_axis output double; blob_orientation output double; blob_eccentricity output double; blob_extent output double; blob_count output double; blob_color output double; bw_image output double
function [blob_hues, blob_area, blob_centroids, blob_bbox, blob_major_axis, blob_minor_axis, blob_orientation, blob_eccentricity, blob_extent, blob_count, blob_color, bw_image] = GetBlobInfo(LabelMatrix, num_colors, ref_colors, ColorFilter, a_range, b_range)
% This function calculates blob information for each color component after
%   iterative segmentation


% Output
%   blob_color = 1xN vector of color indices (global color scheme)


% Initialize
max_num_blobs = 50;
min_blob_area = 5;

[rows, cols] = size(LabelMatrix);
image_area = rows*cols;
LogicMatrix = false(rows,cols);
bw_image = zeros(rows,cols);

blob_hues = zeros(3,max_num_blobs);
blob_area = -1.*ones(1,max_num_blobs);
blob_bbox = zeros(4,max_num_blobs);
blob_major_axis = zeros(1,max_num_blobs);
blob_minor_axis = zeros(1,max_num_blobs);
blob_centroids = zeros(2,max_num_blobs);
blob_eccentricity = zeros(1,max_num_blobs);
blob_extent = zeros(1,max_num_blobs);
blob_orientation = zeros(1,max_num_blobs);
blob_count = 0;

blob_color = zeros(1,max_num_blobs);

max_num_col_filter = length(ColorFilter);
num_col_filter = sum(ColorFilter);

area_thresh = .1;


% Determine L_white and L_black as needed
find_white = 0;
find_black = 0;
L_white = 101;
L_black = -1;
color_areas = zeros(1,size(ref_colors,1));

if(ColorFilter(1) + ColorFilter(2) > 0)
    for row = 1:rows
        for col = 1:cols
            color_areas(LabelMatrix(row,col)) = color_areas(LabelMatrix(row,col)) + 1;
        end
    end
end

if(ColorFilter(1) == 1)
    
    % Determine the brightest colors, but allow a maximum area
    %   ratio of the image to be "white"
    find_white = 1;
    
    positive_area = 0;
    for n = 1:num_colors
        
        maxL = -1;
        k_max = -1;
        for k = 1:num_colors
            L = ref_colors(k,1);
            if(L > maxL && L < L_white)
                maxL = L;
                k_max = k;
            end
        end
        
        positive_area = positive_area + color_areas(k_max);
        if(positive_area/image_area >= area_thresh && n > 1)
            break;
        end
        
        L_white = maxL;
        
    end
end

if(ColorFilter(2) == 1)
    
    % Determine the darkest colors, but allow a maximum area
    %   ratio of the image to be "black"
    find_black = 1;
    
    for row = 1:rows
        for col = 1:cols
            color_areas(LabelMatrix(row,col)) = color_areas(LabelMatrix(row,col)) + 1;
        end
    end
    
    positive_area = 0;
    for n = 1:num_colors
        
        minL = 101;
        k_min = -1;
        for k = 1:num_colors
            L = ref_colors(k,1);
            if(L < minL && L > L_black)
                minL = L;
                k_min = k;
            end
        end
        
        positive_area = positive_area + color_areas(k_min);
        if(positive_area/image_area >= area_thresh && n > 1)
            break;
        end
        
        L_black = minL;
        
    end
end


% Input hblob, a matrix containing [Area, blob_centroids, Eccentricity] for each
% identified blob
persistent hblob
if isempty(hblob)
    hblob = video.BlobAnalysis('AreaOutputPort',true,'CentroidOutputPort',true,...
        'BoundingBoxOutputPort',true,'MajorAxisLengthOutputPort',true,'MinorAxisLengthOutputPort',true,...
        'OrientationOutputPort',true,...
        'EccentricityOutputPort',true,'ExtentOutputPort',true,'NumBlobsOutputPort',true,...
        'MinimumBlobAreaSource','Property','MinimumBlobArea', min_blob_area);
end


% Calculate geometric information about the blobs
%
% LogicMatrix is a binary version of LabelMatrix, with ones at all
%   locations for which color values are k, and zeros everywhere else
%
% Explanation
%   condition1 == 1 causes the k'th color to be analyzed by blob analysis,
%     as well as be included in the black-and-white image
%   condition1 == 0 disallows both of these items and simply ignores color
%     k
%   condition0 == 1 ensures that condition1 is true for all k
%   condition0 == 0 enforces a filter which allows only the colors
%     specified in the ColorFilter vector
condition0 = (num_col_filter == 0);
current_color = 0;
for k = 1:num_colors
    
    % Decide whether or not to perform blob analysis
    condition1 = 0;
    if(condition0)
        condition1 = 1;
    else
        a = ref_colors(k, 2);
        b = ref_colors(k, 3);
        for i = 1:max_num_col_filter
            
            % Skip colors that have not been specified
            if(ColorFilter(i) == 0)
                continue;
            end
            
            if( find_white == 1 && ref_colors(k,1) >= L_white)  % Handle "white" differently than other colors
                condition1 = 1;
                current_color = 1;
                break;
            elseif( find_black == 1 && ref_colors(k,1) <= L_black)  % Handle "black" differently than other colors
                condition1 = 1;
                current_color = 2;
                break;
            elseif( a >= a_range(1,i) && a <= a_range(2,i) && b >= b_range(1,i) && b <= b_range(2,i) )
                condition1 = 1;
                current_color = i;
                break;
            end
            
        end
    end
    
    % Blob analysis
    if( condition1 == 1 )
        
        for i = 1:rows
            for j = 1:cols
                if(LabelMatrix(i,j) ~= k)
                    LogicMatrix(i,j) = false;
                else
                    LogicMatrix(i,j) = true;
                    bw_image(i,j) = 1;
                end
            end
        end

        [TArea,TCentroid,TBBox,TMajorAxis,TMinorAxis,TOrientation,TEccent,TExtent,TNumBlobs] = step(hblob,LogicMatrix);

        for i = 1:TNumBlobs
            if(blob_count + TNumBlobs <= max_num_blobs)

                blob_centroids(1,blob_count+i) = TCentroid(1,i);
                blob_centroids(2,blob_count+i) = TCentroid(2,i);

                ii = round(blob_centroids(1,blob_count+i));
                jj = round(blob_centroids(2,blob_count+i));

                blob_hues(1,blob_count+i) = ref_colors( LabelMatrix(ii,jj), 1 );
                blob_hues(2,blob_count+i) = ref_colors( LabelMatrix(ii,jj), 2 );
                blob_hues(3,blob_count+i) = ref_colors( LabelMatrix(ii,jj), 3 );

                blob_area(blob_count+i) = TArea(i);
                blob_bbox(blob_count+i) = TBBox(i);
                blob_major_axis(blob_count+i) = TMajorAxis(i);
                blob_minor_axis(blob_count+i) = TMinorAxis(i);
                blob_eccentricity(blob_count+i) = TEccent(i);
                blob_extent(blob_count+i) = TExtent(i);
                blob_orientation(blob_count+i) = TOrientation(i);
                
                blob_color(blob_count+i) = current_color;

            end
        end

        blob_count = blob_count + double(TNumBlobs);

    end
    
end


return

== matlab function Transform Coordinates2 ==
  data: bw_image_in input double; which_camera input double; x_in input double; y_in input double; r_out output double; c_out output double; z_in input double
function [r_out, c_out] = transform_G2L(bw_image_in, which_camera, x_in, y_in, z_in)
% This function, "transform Global to Local coordinates," transforms
%   global coordinates that are sent to the controller into local
%   coordinates that can be displayed over images.
%
% 5-29-11
%
% Input
%   x_in, y_in, z_in = vectors of points in global (vehicle-centered)
%     coordinate system
%   bw_image_in = a 2-D array of pixel values (used only to extract image
%     size)
%   which_camera = selects which camera for relative coordinates
%                = 0 -> Forward camera
%                = 1 -> Down camera
%
% Output
%   r_out, c_out = row, column pairs in local coordinate system

[rows, cols] = size(bw_image_in);
if( which_camera == 0 )
    r_out = z_in + floor(rows/2);
    c_out = y_in + floor(cols/2);
else
    r_out = floor(rows/2) - x_in;
    c_out = y_in + floor(cols/2);
end

return

== matlab function Blob_Analysis/Blob_Analysis1/IterativeSegmentation/Low Pass Filter/Low Pass Filter ==
  data: I input double; Iout output double
function Iout = GaussianBlurr(I)
% This function calculates the gaussian blur of an intensity image

sigma = sqrt(2);

Grows = 3;    % Gaussian matrix rows
Gcols = 3;    % Gaussian matrix columns

[Irows Icols] = size(I);

Iout = double(zeros(Irows,Icols));

Trows = Irows - Grows + 1;
Tcols = Icols - Gcols + 1;
Itemp = double(zeros(Trows,Tcols));

G = zeros(Grows,Gcols);

FirstRow = ceil(-Grows/2);
LastRow = floor(Grows/2);
FirstCol = ceil(-Gcols/2);
LastCol = floor(Gcols/2);
Gsum = 0;
for i=FirstRow:LastRow
    for j = FirstCol:LastCol
        G(i-FirstRow+1,j-FirstCol+1) = exp(-(j*j+i*i)/(2*sigma*sigma));
        Gsum = Gsum + G(i-FirstRow+1,j-FirstCol+1);
    end
end

G = G./Gsum;

Itemp = conv2(double(I),double(G),'valid');

% reflect boundaries to keep image the same size
% top
Iout((1:LastRow),(LastCol+1:Icols-LastCol)) = Itemp((1:LastRow),(1:Tcols));
% bottom
Iout((Irows-LastRow+1:Irows),(LastCol+1:Icols-LastCol)) = Itemp((Trows-LastRow+1:Trows),(1:Tcols));
% left
Iout((1+LastRow:Irows-LastRow),(1:LastCol)) = Itemp((1:Trows),(1:LastCol));
% right
Iout((1+LastRow:Irows-LastRow),(Icols-LastCol+1:Icols)) = Itemp((1:Trows),(Tcols-LastCol+1:Tcols));
% center
Iout((1+LastRow:Irows-LastRow),(1+LastCol:Icols-LastCol)) = Itemp;
% top left corner
Iout(1:LastRow,1:LastCol) = Itemp(1:LastRow,1:LastCol);
% top right corner
Iout(1:LastRow,Icols-LastCol:Icols) = Itemp(1:LastRow,Tcols-LastCol:Tcols);
% bottom left corner
Iout(Irows-LastRow:Irows,1:LastCol) = Itemp(Trows-LastRow:Trows,1:LastCol);
% bottom right corner
Iout(Irows-LastRow:Irows,Icols-LastCol:Icols) = Itemp(Trows-LastRow:Trows,Tcols-LastCol:Tcols);

return

== matlab function Blob_Analysis/Blob_Analysis1/IterativeSegmentation/Low Pass Filter/Low Pass Filter1 ==
  data: I input double; Iout output double
function Iout = GaussianBlurr(I)
% This function calculates the gaussian blur of an intensity image

sigma = sqrt(2);

Grows = 3;    % Gaussian matrix rows
Gcols = 3;    % Gaussian matrix columns

[Irows Icols] = size(I);

Iout = double(zeros(Irows,Icols));

Trows = Irows - Grows + 1;
Tcols = Icols - Gcols + 1;
Itemp = double(zeros(Trows,Tcols));

G = zeros(Grows,Gcols);

FirstRow = ceil(-Grows/2);
LastRow = floor(Grows/2);
FirstCol = ceil(-Gcols/2);
LastCol = floor(Gcols/2);
Gsum = 0;
for i=FirstRow:LastRow
    for j = FirstCol:LastCol
        G(i-FirstRow+1,j-FirstCol+1) = exp(-(j*j+i*i)/(2*sigma*sigma));
        Gsum = Gsum + G(i-FirstRow+1,j-FirstCol+1);
    end
end

G = G./Gsum;

Itemp = conv2(double(I),double(G),'valid');

% reflect boundaries to keep image the same size
% top
Iout((1:LastRow),(LastCol+1:Icols-LastCol)) = Itemp((1:LastRow),(1:Tcols));
% bottom
Iout((Irows-LastRow+1:Irows),(LastCol+1:Icols-LastCol)) = Itemp((Trows-LastRow+1:Trows),(1:Tcols));
% left
Iout((1+LastRow:Irows-LastRow),(1:LastCol)) = Itemp((1:Trows),(1:LastCol));
% right
Iout((1+LastRow:Irows-LastRow),(Icols-LastCol+1:Icols)) = Itemp((1:Trows),(Tcols-LastCol+1:Tcols));
% center
Iout((1+LastRow:Irows-LastRow),(1+LastCol:Icols-LastCol)) = Itemp;
% top left corner
Iout(1:LastRow,1:LastCol) = Itemp(1:LastRow,1:LastCol);
% top right corner
Iout(1:LastRow,Icols-LastCol:Icols) = Itemp(1:LastRow,Tcols-LastCol:Tcols);
% bottom left corner
Iout(Irows-LastRow:Irows,1:LastCol) = Itemp(Trows-LastRow:Trows,1:LastCol);
% bottom right corner
Iout(Irows-LastRow:Irows,Icols-LastCol:Icols) = Itemp(Trows-LastRow:Trows,Tcols-LastCol:Tcols);

return

== matlab function Blob_Analysis/Blob_Analysis1/IterativeSegmentation/Low Pass Filter/Low Pass Filter2 ==
  data: I input double; Iout output double
function Iout = GaussianBlurr(I)
% This function calculates the gaussian blur of an intensity image

sigma = sqrt(2);

Grows = 3;    % Gaussian matrix rows
Gcols = 3;    % Gaussian matrix columns

[Irows Icols] = size(I);

Iout = double(zeros(Irows,Icols));

Trows = Irows - Grows + 1;
Tcols = Icols - Gcols + 1;
Itemp = double(zeros(Trows,Tcols));

G = zeros(Grows,Gcols);

FirstRow = ceil(-Grows/2);
LastRow = floor(Grows/2);
FirstCol = ceil(-Gcols/2);
LastCol = floor(Gcols/2);
Gsum = 0;
for i=FirstRow:LastRow
    for j = FirstCol:LastCol
        G(i-FirstRow+1,j-FirstCol+1) = exp(-(j*j+i*i)/(2*sigma*sigma));
        Gsum = Gsum + G(i-FirstRow+1,j-FirstCol+1);
    end
end

G = G./Gsum;

Itemp = conv2(double(I),double(G),'valid');

% reflect boundaries to keep image the same size
% top
Iout((1:LastRow),(LastCol+1:Icols-LastCol)) = Itemp((1:LastRow),(1:Tcols));
% bottom
Iout((Irows-LastRow+1:Irows),(LastCol+1:Icols-LastCol)) = Itemp((Trows-LastRow+1:Trows),(1:Tcols));
% left
Iout((1+LastRow:Irows-LastRow),(1:LastCol)) = Itemp((1:Trows),(1:LastCol));
% right
Iout((1+LastRow:Irows-LastRow),(Icols-LastCol+1:Icols)) = Itemp((1:Trows),(Tcols-LastCol+1:Tcols));
% center
Iout((1+LastRow:Irows-LastRow),(1+LastCol:Icols-LastCol)) = Itemp;
% top left corner
Iout(1:LastRow,1:LastCol) = Itemp(1:LastRow,1:LastCol);
% top right corner
Iout(1:LastRow,Icols-LastCol:Icols) = Itemp(1:LastRow,Tcols-LastCol:Tcols);
% bottom left corner
Iout(Irows-LastRow:Irows,1:LastCol) = Itemp(Trows-LastRow:Trows,1:LastCol);
% bottom right corner
Iout(Irows-LastRow:Irows,Icols-LastCol:Icols) = Itemp(Trows-LastRow:Trows,Tcols-LastCol:Tcols);

return
